simulink model "motor"  (R2016b)
settings: Solver=ode15s  StartTime=0.0  StopTime=10.0  RelTol=1e-3
values from neighbouring files (symbols this model uses):
  b = 0.0167    [script.m]
  J = 0.0167    [script.m]
  Kb = 0.8    [script.m]
  Kt = 0.8    [script.m]
  La = 0.012    [script.m]
  Ra = 0.6    [script.m]
libraries: simulink x1
settings Model: Creator=Daniel  LastModifiedBy=Daniel

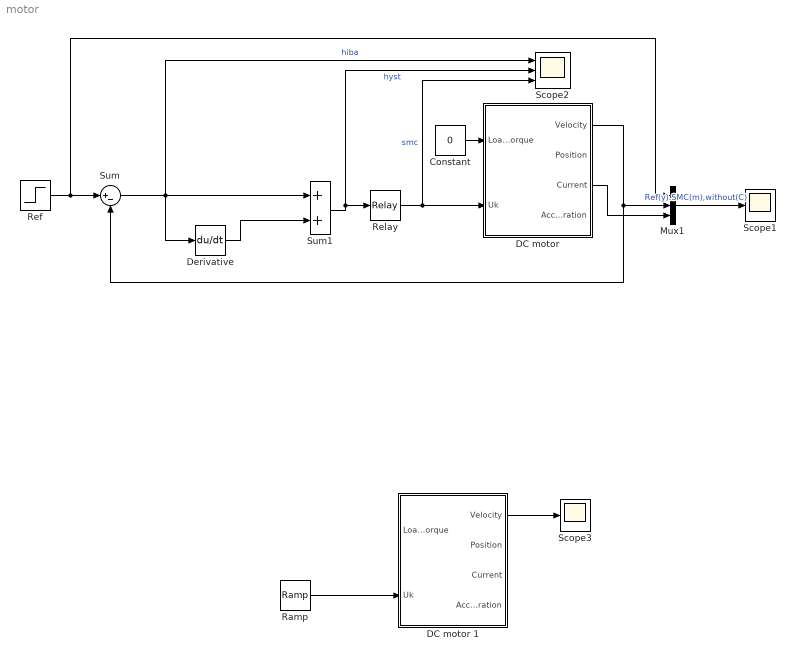
== system motor ==
  Constant : Constant  Value=0
  "DC motor " : Subsystem
  DC motor 1 : Subsystem
  Derivative : Derivative  CoefficientInTFapproximation=0.01
  Mux1 : Mux  Inputs=3
  Ramp : simulink/Sources/Ramp  slope=1  start=0  X0=0
  Ref : Step  SampleTime=0
  Relay : Relay  OnSwitchValue=0.1  OffSwitchValue=-0.1  OnOutputValue=10  OffOutputValue=-10
  Scope1 : Scope
  Scope2 : Scope  NumInputPorts=3
  Scope3 : Scope
  Sum : Sum  Inputs=|+-
  Sum1 : Sum
  wires:
  Sum1/1 -> Scope2/2, Relay/1  "hyst"
  Derivative/1 -> Sum1/2
  Sum/1 -> Sum1/1, Scope2/1, Derivative/1  "hiba"
  Ref/1 -> Sum/1, Mux1/1
  Mux1/1 -> Scope1/1  "Ref(y).SMC(m),without(C)"
  Relay/1 -> "DC motor "/2("Uk "), Scope2/3  "smc"
  Constant/1 -> "DC motor "/1(Load Torque)
  "DC motor "/1("Velocity ") -> Sum/2, Mux1/2
  "DC motor "/3(Current) -> Mux1/3
  Ramp/1 -> DC motor 1/2("Uk ")
  DC motor 1/1("Velocity ") -> Scope3/1

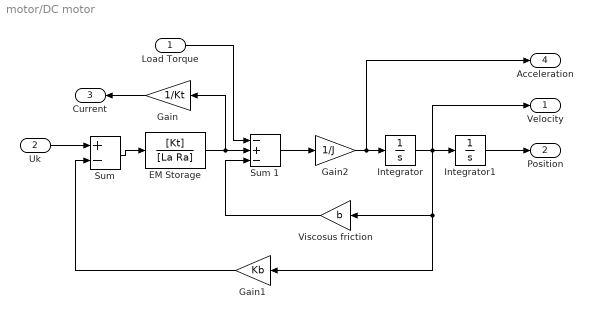
== system motor/DC motor  ==
  Load Torque : Inport
  "Uk " : Inport  Port=2  Interpolate=off
  "EM Storage " : TransferFcn  Numerator=[Kt]  Denominator=[La Ra]
  Gain : Gain  Gain=1/Kt
  Gain1 : Gain  Gain=Kb
  Gain2 : Gain  Gain=1/J
  Integrator : Integrator
  Integrator1 : Integrator
  "Sum " : Sum  Inputs=+-
  Sum 1 : Sum  Inputs=-+-
  Viscosus friction : Gain  Gain=b
  "Velocity " : Outport
  Position : Outport  Port=2
  Current : Outport  Port=3
  Acceleration : Outport  Port=4
  wires:
  Viscosus friction/1 -> Sum 1/3
  Integrator/1 -> "Velocity "/1, Gain1/1, Viscosus friction/1, Integrator1/1
  Integrator1/1 -> Position/1
  "EM Storage "/1 -> Gain/1, Sum 1/2
  Gain/1 -> Current/1
  Load Torque/1 -> Sum 1/1
  Gain2/1 -> Acceleration/1, Integrator/1
  Sum 1/1 -> Gain2/1
  "Sum "/1 -> "EM Storage "/1
  "Uk "/1 -> "Sum "/1
  Gain1/1 -> "Sum "/2

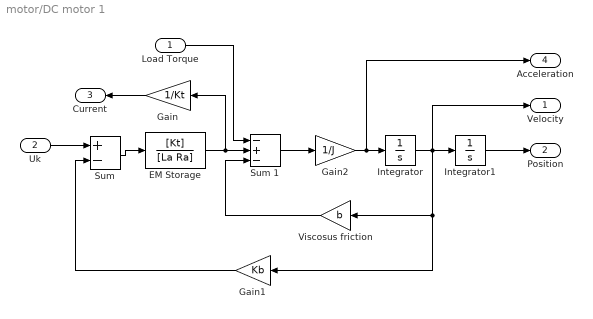
== system motor/DC motor 1 ==
  Load Torque : Inport
  "Uk " : Inport  Port=2  Interpolate=off
  "EM Storage " : TransferFcn  Numerator=[Kt]  Denominator=[La Ra]
  Gain : Gain  Gain=1/Kt
  Gain1 : Gain  Gain=Kb
  Gain2 : Gain  Gain=1/J
  Integrator : Integrator
  Integrator1 : Integrator
  "Sum " : Sum  Inputs=+-
  Sum 1 : Sum  Inputs=-+-
  Viscosus friction : Gain  Gain=b
  "Velocity " : Outport
  Position : Outport  Port=2
  Current : Outport  Port=3
  Acceleration : Outport  Port=4
  wires:
  Viscosus friction/1 -> Sum 1/3
  Integrator/1 -> "Velocity "/1, Gain1/1, Viscosus friction/1, Integrator1/1
  Integrator1/1 -> Position/1
  "EM Storage "/1 -> Gain/1, Sum 1/2
  Gain/1 -> Current/1
  Load Torque/1 -> Sum 1/1
  Gain2/1 -> Acceleration/1, Integrator/1
  Sum 1/1 -> Gain2/1
  "Sum "/1 -> "EM Storage "/1
  "Uk "/1 -> "Sum "/1
  Gain1/1 -> "Sum "/2
